simulink model "data_parametric_model_block"  (R2014a)
settings: Solver=ode45  StartTime=0.0  StopTime=10.0  RelTol=1e-3
PostLoadFcn:
  | % Import the data from Excel for a lookup table
  | data = xlsread('thrust_curve','Sheet1');
  | % Row indices for lookup table
  | breakpoints1 = data(2:end,1)';
  | % Column indices for lookup table
  | breakpoints2 = data(1,2:end);
  | % Output values for lookup table
  | table_data = data(2:end,2:end);
settings Model: Creator=scorpii  LastModifiedBy=scorpii
settings OptimizationCC: BlockReduction=off  InlineParams=on  BufferReuse=off  SimCompilerOptimization=off
settings DebuggingCC: MergeDetectMultiDrivingBlocksExec=error  FrameProcessingCompatibilityMsg=error
settings RTWCC: RTWCompilerOptimization=off

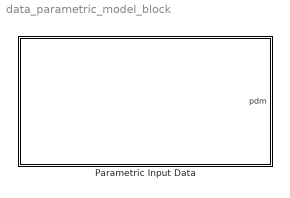
== system data_parametric_model_block ==
  Parametric Input Data : Subsystem

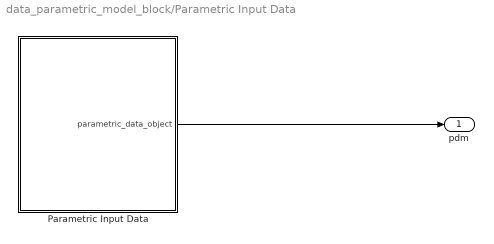
== system data_parametric_model_block/Parametric Input Data ==
  Parametric Input Data : MATLAB Function  TreatAsAtomicUnit=on
  pdm : Outport
  wires:
  Parametric Input Data/1(parametric_data_object) -> pdm/1

== matlab function data_parametric_model_block/User-Defined Functions/MATLAB Function ==
  data: u input; y output
function y = fcn(u)
%#codegen

y = u;

== matlab function data_parametric_model_block/Air Density ==
  data: T_in input; rho output; P_in input; alt_in input
function rho = ISA_model(T_in, P_in, alt_in)

% This model computes the gas characteristics of the atmosphere around the
% rocket based on temperature and pressure at launch and current altitude.
% It uses the International Standard Atmosphere (ISA) model. This model is 
% only effective BELOW the tropopause.

% Model is based on the following document:
%   http://home.anadolu.edu.tr/~mcavcar/common/ISAweb.pdf

% Define required constants for the model as per ISA mean sea-level
% conditions:
%   P_o     = standard pressure (Pascals)
%   T_o     = standard temperature (degrees K)
%   R       = gas Constants (m^2/K*s^2)

    P_o     = 101325;
    T_o     = 288.15;
    R       = 287.04;
    
% The following recalculates the temperature in terms of ISA deviation.
% Variables used:
%   T_dev   = ISA deviation temperature (degrees C)
%   T_in    = ground temperature (degrees C)

    T_dev   = T_in - T_o + 273.15;
    
% The following calculates the temperature at the current altitude.
% Variables used:
%   T_act   = Actual temperature at current altitude (degrees K)
%   alt_in  = Actual altitude (m)

    T_act   = (T_o + T_dev) - (6.5/1000)*alt_in;
    
% The following recalculates the pressure in terms of ISA deviation.
% Variables used:
%   P_dev   = ISA deviation pressure (Pascals)
%   P_in    = ground pressure (Pascals)

    P_dev   = P_in - P_o;
    
% The following calculates the ambient pressure at the current altitude.
% Variables used:
%   P_act   = actual pressure at current altitude (Pascals)

    P_act   = (P_o + P_dev)*((1 - 0.0065*(alt_in/(T_o + T_dev)))^5.2561);
    
% The following calculates the air density at the current altitude.
% Variables used:
%   rho = air density at current altitude (Kg/m^3)

    rho = P_act/(R*T_act);
    
% END OF FUNCTION

== matlab function data_parametric_model_block/Parametric Input Data/Parametric Input Data ==
  data: parametric_data_object output
function parametric_data_object = data_parametric_model()
%--------------------------------------------------------------------------------
%
% data_parametric_model.m
%
% Data Access of Parametric Model
%
% Design Parameters for the Rocket are stored in a spreadsheet. 
% These parameters will be accessed and passed along into the simulation to 
% determine other parameters and ultimately to evaluate the performance of 
% those design values
%
%--------------------------------------------------------------------------------
% References
% http://www.mathworks.com/help/simulink/ug/how-to-import-data-from-an-excel-spreadsheet.html
% http://www.mathworks.com/help/matlab/matlab_external/example-reading-excel-spreadsheet-data.html
%--------------------------------------------------------------------------------

% Import the data from Excel
% data = xlsread('input_parameters.csv','B2:B23');
spreadsheet_data = xlsread('Parametric_Data.xlsm','Matlab_Data','B2:B23');

% set keyset to store keys which will map values for parametric parameters

keyset = {'area_fin_frontal', 'area_face_fin', 'width_fins_at_tube', 'fins_count', 'thickness_fins_at_tube', 'area_surface_nose', 'height_fins', 'diameter_outer', 'surface_roughness', 'length_total_rocket', 'pressure_ambient_ground', 'temperature_ambient_ground', 'edge_rounding', 'distance_tip_to_COG', 'distance_tip_to_COP', 'angle_leading_edge', 'fin_leading_edge_profile', 'fin_trailing_edge_profile', 'diameter_outer_launch_guide', 'diameter_inner_launch_guide', 'moment_inertia_rocket'};

valueset = {0, 0, 0, 0, 0, 0, 0, 0, 0, 0, 0, 0, 0, 0, 0, 0, 0, 0, 0, 0, 0};

% initialize map object to store parametric data
parametric_data_object = containers.Map(keyset,valueset)

% Extract parameters from the imported data file
parametric_data_object('area_fin_frontal')            = spreadsheet_data(1,1)
parametric_data_object('area_face_fin')               = spreadsheet_data(2,1)
parametric_data_object('width_fins_at_tube')          = spreadsheet_data(3,1)
parametric_data_object('fins_count')                  = spreadsheet_data(4,1)
parametric_data_object('thickness_fins_at_tube')      = spreadsheet_data(5,1)
parametric_data_object('area_surface_nose')           = spreadsheet_data(6,1)
parametric_data_object('height_fins')                 = spreadsheet_data(7,1)
parametric_data_object('diameter_outer')              = spreadsheet_data(8,1)
parametric_data_object('surface_roughness')           = spreadsheet_data(9,1)
parametric_data_object('length_total_rocket')         = spreadsheet_data(10,1)
parametric_data_object('pressure_ambient_ground')     = spreadsheet_data(11,1)
parametric_data_object('temperature_ambient_ground')  = spreadsheet_data(12,1)
parametric_data_object('edge_rounding')               = spreadsheet_data(13,1)
parametric_data_object('distance_tip_to_COG')         = spreadsheet_data(14,1)
parametric_data_object('distance_tip_to_COP')         = spreadsheet_data(15,1)
parametric_data_object('angle_leading_edge')          = spreadsheet_data(16,1)
parametric_data_object('fin_leading_edge_profile')    = spreadsheet_data(17,1)
parametric_data_object('fin_trailing_edge_profile')   = spreadsheet_data(18,1)
parametric_data_object('diameter_outer_launch_guide') = spreadsheet_data(19,1)
parametric_data_object('diameter_inner_launch_guide') = spreadsheet_data(20,1)
parametric_data_object('moment_inertia_rocket')       = spreadsheet_data(21,1)

end
